simulink model "model_sim_CHB9"  (R2023b)
settings: Solver=FixedStepAuto  StartTime=0.0  StopTime=5  FixedStep=1e-6  RelTol=1e-3
InitFcn:
  | sysinit
values from neighbouring files (symbols this model uses):
  C = 0.0234    [sysinit.m]
  f = 50    [sysinit.m]
  f_switch = 250    [sysinit.m]
  fn = 50    [sysinit.m]
  L = 0.002    [sysinit.m]
  L_ori = 0.02    [sysinit.m]
  L_sec = 0.06    [sysinit.m]
  m = 0.95    [sysinit.m]
  P0 = 8e6    (= 8000000)    [sysinit.m]
  R = 1.5    [sysinit.m]
  Source_Amp = 10000    [sysinit.m]
  st = 1e-6    (= 1e-06)    [sysinit.m]
  Td = 15e-7    (= 1.5e-06)    [sysinit.m]
  Ul_in = 1900    [sysinit.m]
libraries: spsSeriesRLCBranchLib x123, spsDiodeLib x60, spsIGBTLib x48, spsCurrentMeasurementLib x16, spsThreePhaseVIMeasurementLib x13, spsOnDelayLib x12, spsUniversalBridgeLib x12, spsMultiWindingTransformerLib x9, simulink x3, spsVoltageMeasurementLib x3, spsRMSLib x2, spsThreePhaseProgrammableVoltageSourceLib x1
(part 2 of 3)

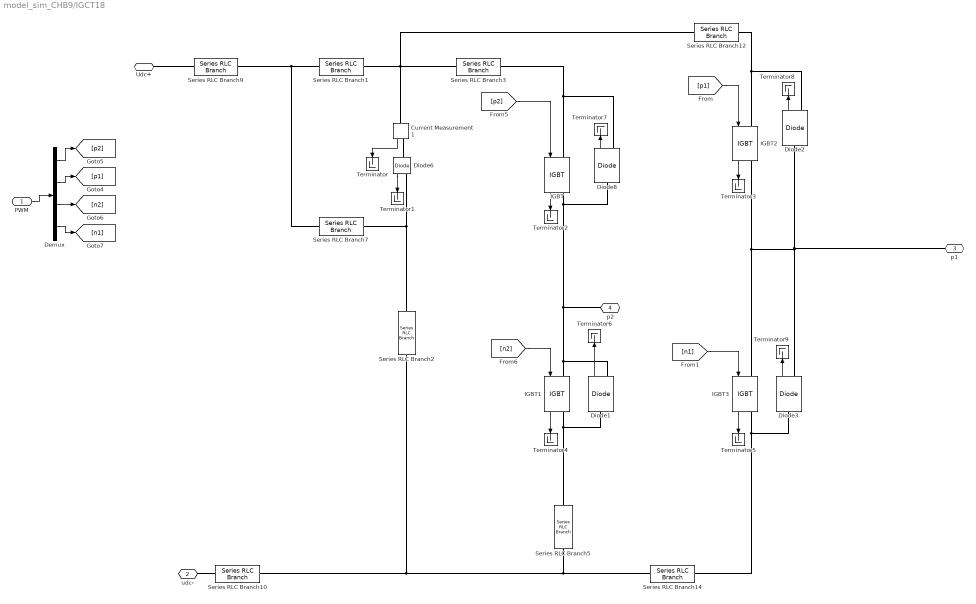
== system model_sim_CHB9/IGCT18 ==
  PWM : Inport
  Current Measurement1 : spsCurrentMeasurementLib/Current Measurement  PhasorSimulation=off  OutputType=Complex  PSBequivalent=0
  Demux : Demux
  Diode{1..3,6,8} (5 alike) : spsDiodeLib/Diode  Ron=rto  Lon=0  Vf=vto  IC=0  UseSnubber=off  Rs=500  Cs=250e-9  Measurements=on
  IGBT{,1..3} (4 alike) : spsIGBTLib/IGBT  Ron=rt  Lon=0  Vf=vt  Tf=1e-6  Tt=2e-6  IC=0  Rs=1e5  Cs=inf  Measurements=on
  Series RLC Branch1 : spsSeriesRLCBranchLib/Series RLC Branch  LConnTagsString=__new0  RConnTagsString=__new0  BranchType=RL  Resistance=1e-5  Inductance=3.0E-6  SetiL0=off  InitialCurrent=0  Capacitance=1e-6  Setx0=off  InitialVoltage=0  Measurements=None
  Series RLC Branch10 : spsSeriesRLCBranchLib/Series RLC Branch  LConnTagsString=__new0  RConnTagsString=__new0  BranchType=L  Resistance=1  Inductance=0.4e-6  SetiL0=off  InitialCurrent=0  Capacitance=1e-6  Setx0=off  InitialVoltage=0  Measurements=None
  Series RLC Branch12 : spsSeriesRLCBranchLib/Series RLC Branch  LConnTagsString=__new0  RConnTagsString=__new0  BranchType=RL  Resistance=1e-5  Inductance=1E-9  SetiL0=off  InitialCurrent=0  Capacitance=1e-6  Setx0=off  InitialVoltage=0  Measurements=None
  Series RLC Branch14 : spsSeriesRLCBranchLib/Series RLC Branch  LConnTagsString=__new0  RConnTagsString=__new0  BranchType=L  Resistance=1  Inductance=1E-7  SetiL0=off  InitialCurrent=0  Capacitance=1e-6  Setx0=off  InitialVoltage=0  Measurements=None
  Series RLC Branch2 : spsSeriesRLCBranchLib/Series RLC Branch  LConnTagsString=__new0  RConnTagsString=__new0  BranchType=RC  Resistance=1e-5  Inductance=20e-6  SetiL0=off  InitialCurrent=0  Capacitance=17e-6  Setx0=off  InitialVoltage=0  Measurements=None
  Series RLC Branch3 : spsSeriesRLCBranchLib/Series RLC Branch  LConnTagsString=__new0  RConnTagsString=__new0  BranchType=RL  Resistance=1e-5  Inductance=1E-9  SetiL0=off  InitialCurrent=0  Capacitance=1e-6  Setx0=off  InitialVoltage=0  Measurements=None
  Series RLC Branch5 : spsSeriesRLCBranchLib/Series RLC Branch  LConnTagsString=__new0  RConnTagsString=__new0  BranchType=L  Resistance=1  Inductance=1E-7  SetiL0=off  InitialCurrent=0  Capacitance=1e-6  Setx0=off  InitialVoltage=0  Measurements=None
  Series RLC Branch7 : spsSeriesRLCBranchLib/Series RLC Branch  LConnTagsString=__new0  RConnTagsString=__new0  BranchType=RL  Resistance=0.6  Inductance=1e-6  SetiL0=off  InitialCurrent=0  Capacitance=1e-6  Setx0=off  InitialVoltage=0  Measurements=None
  Series RLC Branch9 : spsSeriesRLCBranchLib/Series RLC Branch  LConnTagsString=__new0  RConnTagsString=__new0  BranchType=L  Resistance=1  Inductance=0.4e-6  SetiL0=off  InitialCurrent=0  Capacitance=1e-6  Setx0=off  InitialVoltage=0  Measurements=None
  Terminator{,1..9} (10 alike) : Terminator
  Udc+ : PMIOPort  Side=Left
  udc- : PMIOPort  Port=2  Side=Left
  p1 : PMIOPort  Port=3  Side=Right
  p2 : PMIOPort  Port=4  Side=Right
  wires:
  Diode3/1 -> Terminator9/1
  IGBT3/1 -> Terminator5/1
  [n1] -> IGBT3/1
  IGBT1/1 -> Terminator4/1
  IGBT2/1 -> Terminator3/1
  IGBT/1 -> Terminator2/1
  [n2] -> IGBT1/1
  [p1] -> IGBT2/1
  Current Measurement1/1 -> Terminator/1
  Diode2/1 -> Terminator8/1
  [p2] -> IGBT/1
  Diode8/1 -> Terminator7/1
  Diode1/1 -> Terminator6/1
  Diode6/1 -> Terminator1/1
  Demux/3 -> [n2]
  PWM/1 -> Demux/1
  Demux/1 -> [p2]
  Demux/2 -> [p1]
  Demux/4 -> [n1]
  connections:
  Series RLC Branch10/LConn1 -- udc-/RConn1
  Series RLC Branch9/LConn1 -- Udc+/RConn1
  Diode6/RConn1 -- Series RLC Branch7/RConn1 -- Series RLC Branch2/LConn1
  Current Measurement1/LConn1 -- Series RLC Branch1/RConn1 -- Series RLC Branch3/LConn1 -- Series RLC Branch12/LConn1
  Diode3/LConn1 -- IGBT3/RConn1 -- Series RLC Branch14/RConn1
  Series RLC Branch3/RConn1 -- IGBT/LConn1 -- Diode8/RConn1
  Diode1/LConn1 -- Series RLC Branch5/RConn1 -- IGBT1/RConn1
  Current Measurement1/RConn1 -- Diode6/LConn1
  Diode2/RConn1 -- Series RLC Branch12/RConn1 -- IGBT2/LConn1
  p1/RConn1 -- Diode2/LConn1 -- Diode3/RConn1 -- IGBT3/LConn1 -- IGBT2/RConn1
  Series RLC Branch5/LConn1 -- Series RLC Branch14/LConn1 -- Series RLC Branch10/RConn1 -- Series RLC Branch2/RConn1
  Series RLC Branch1/LConn1 -- Series RLC Branch7/LConn1 -- Series RLC Branch9/RConn1
  p2/RConn1 -- IGBT1/LConn1 -- Diode1/RConn1 -- Diode8/LConn1 -- IGBT/RConn1

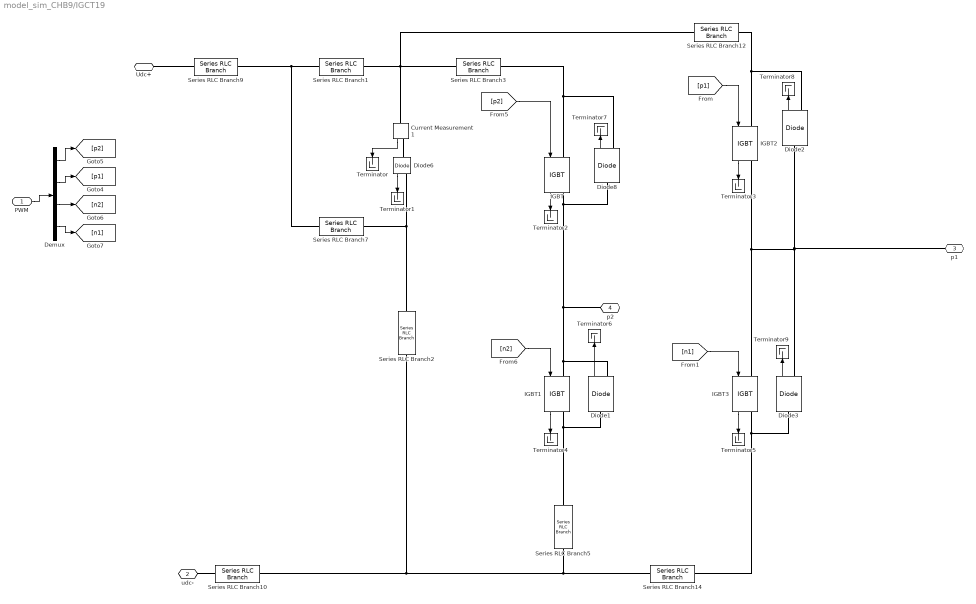
== system model_sim_CHB9/IGCT19 ==
  PWM : Inport
  Current Measurement1 : spsCurrentMeasurementLib/Current Measurement  PhasorSimulation=off  OutputType=Complex  PSBequivalent=0
  Demux : Demux
  Diode{1..3,6,8} (5 alike) : spsDiodeLib/Diode  Ron=rto  Lon=0  Vf=vto  IC=0  UseSnubber=off  Rs=500  Cs=250e-9  Measurements=on
  IGBT{,1..3} (4 alike) : spsIGBTLib/IGBT  Ron=rt  Lon=0  Vf=vt  Tf=1e-6  Tt=2e-6  IC=0  Rs=1e5  Cs=inf  Measurements=on
  Series RLC Branch1 : spsSeriesRLCBranchLib/Series RLC Branch  LConnTagsString=__new0  RConnTagsString=__new0  BranchType=RL  Resistance=1e-5  Inductance=3.0E-6  SetiL0=off  InitialCurrent=0  Capacitance=1e-6  Setx0=off  InitialVoltage=0  Measurements=None
  Series RLC Branch10 : spsSeriesRLCBranchLib/Series RLC Branch  LConnTagsString=__new0  RConnTagsString=__new0  BranchType=L  Resistance=1  Inductance=0.4e-6  SetiL0=off  InitialCurrent=0  Capacitance=1e-6  Setx0=off  InitialVoltage=0  Measurements=None
  Series RLC Branch12 : spsSeriesRLCBranchLib/Series RLC Branch  LConnTagsString=__new0  RConnTagsString=__new0  BranchType=RL  Resistance=1e-5  Inductance=1E-9  SetiL0=off  InitialCurrent=0  Capacitance=1e-6  Setx0=off  InitialVoltage=0  Measurements=None
  Series RLC Branch14 : spsSeriesRLCBranchLib/Series RLC Branch  LConnTagsString=__new0  RConnTagsString=__new0  BranchType=L  Resistance=1  Inductance=1E-7  SetiL0=off  InitialCurrent=0  Capacitance=1e-6  Setx0=off  InitialVoltage=0  Measurements=None
  Series RLC Branch2 : spsSeriesRLCBranchLib/Series RLC Branch  LConnTagsString=__new0  RConnTagsString=__new0  BranchType=RC  Resistance=1e-5  Inductance=20e-6  SetiL0=off  InitialCurrent=0  Capacitance=17e-6  Setx0=off  InitialVoltage=0  Measurements=None
  Series RLC Branch3 : spsSeriesRLCBranchLib/Series RLC Branch  LConnTagsString=__new0  RConnTagsString=__new0  BranchType=RL  Resistance=1e-5  Inductance=1E-9  SetiL0=off  InitialCurrent=0  Capacitance=1e-6  Setx0=off  InitialVoltage=0  Measurements=None
  Series RLC Branch5 : spsSeriesRLCBranchLib/Series RLC Branch  LConnTagsString=__new0  RConnTagsString=__new0  BranchType=L  Resistance=1  Inductance=1E-7  SetiL0=off  InitialCurrent=0  Capacitance=1e-6  Setx0=off  InitialVoltage=0  Measurements=None
  Series RLC Branch7 : spsSeriesRLCBranchLib/Series RLC Branch  LConnTagsString=__new0  RConnTagsString=__new0  BranchType=RL  Resistance=0.6  Inductance=1e-6  SetiL0=off  InitialCurrent=0  Capacitance=1e-6  Setx0=off  InitialVoltage=0  Measurements=None
  Series RLC Branch9 : spsSeriesRLCBranchLib/Series RLC Branch  LConnTagsString=__new0  RConnTagsString=__new0  BranchType=L  Resistance=1  Inductance=0.4e-6  SetiL0=off  InitialCurrent=0  Capacitance=1e-6  Setx0=off  InitialVoltage=0  Measurements=None
  Terminator{,1..9} (10 alike) : Terminator
  Udc+ : PMIOPort  Side=Left
  udc- : PMIOPort  Port=2  Side=Left
  p1 : PMIOPort  Port=3  Side=Right
  p2 : PMIOPort  Port=4  Side=Right
  wires:
  Diode3/1 -> Terminator9/1
  IGBT3/1 -> Terminator5/1
  [n1] -> IGBT3/1
  IGBT1/1 -> Terminator4/1
  IGBT2/1 -> Terminator3/1
  IGBT/1 -> Terminator2/1
  [n2] -> IGBT1/1
  [p1] -> IGBT2/1
  Current Measurement1/1 -> Terminator/1
  Diode2/1 -> Terminator8/1
  [p2] -> IGBT/1
  Diode8/1 -> Terminator7/1
  Diode1/1 -> Terminator6/1
  Diode6/1 -> Terminator1/1
  Demux/3 -> [n2]
  PWM/1 -> Demux/1
  Demux/1 -> [p2]
  Demux/2 -> [p1]
  Demux/4 -> [n1]
  connections:
  Series RLC Branch10/LConn1 -- udc-/RConn1
  Series RLC Branch9/LConn1 -- Udc+/RConn1
  Diode6/RConn1 -- Series RLC Branch7/RConn1 -- Series RLC Branch2/LConn1
  Current Measurement1/LConn1 -- Series RLC Branch1/RConn1 -- Series RLC Branch3/LConn1 -- Series RLC Branch12/LConn1
  Diode3/LConn1 -- IGBT3/RConn1 -- Series RLC Branch14/RConn1
  Series RLC Branch3/RConn1 -- IGBT/LConn1 -- Diode8/RConn1
  Diode1/LConn1 -- Series RLC Branch5/RConn1 -- IGBT1/RConn1
  Current Measurement1/RConn1 -- Diode6/LConn1
  Diode2/RConn1 -- Series RLC Branch12/RConn1 -- IGBT2/LConn1
  p1/RConn1 -- Diode2/LConn1 -- Diode3/RConn1 -- IGBT3/LConn1 -- IGBT2/RConn1
  Series RLC Branch5/LConn1 -- Series RLC Branch14/LConn1 -- Series RLC Branch10/RConn1 -- Series RLC Branch2/RConn1
  Series RLC Branch1/LConn1 -- Series RLC Branch7/LConn1 -- Series RLC Branch9/RConn1
  p2/RConn1 -- IGBT1/LConn1 -- Diode1/RConn1 -- Diode8/LConn1 -- IGBT/RConn1

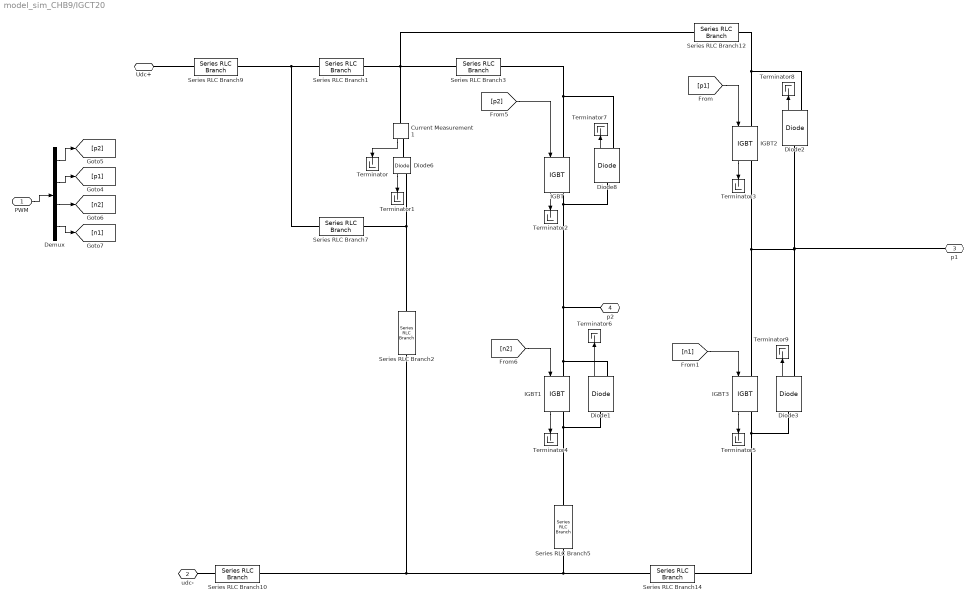
== system model_sim_CHB9/IGCT20 ==
  PWM : Inport
  Current Measurement1 : spsCurrentMeasurementLib/Current Measurement  PhasorSimulation=off  OutputType=Complex  PSBequivalent=0
  Demux : Demux
  Diode{1..3,6,8} (5 alike) : spsDiodeLib/Diode  Ron=rto  Lon=0  Vf=vto  IC=0  UseSnubber=off  Rs=500  Cs=250e-9  Measurements=on
  IGBT{,1..3} (4 alike) : spsIGBTLib/IGBT  Ron=rt  Lon=0  Vf=vt  Tf=1e-6  Tt=2e-6  IC=0  Rs=1e5  Cs=inf  Measurements=on
  Series RLC Branch1 : spsSeriesRLCBranchLib/Series RLC Branch  LConnTagsString=__new0  RConnTagsString=__new0  BranchType=RL  Resistance=1e-5  Inductance=3.0E-6  SetiL0=off  InitialCurrent=0  Capacitance=1e-6  Setx0=off  InitialVoltage=0  Measurements=None
  Series RLC Branch10 : spsSeriesRLCBranchLib/Series RLC Branch  LConnTagsString=__new0  RConnTagsString=__new0  BranchType=L  Resistance=1  Inductance=0.4e-6  SetiL0=off  InitialCurrent=0  Capacitance=1e-6  Setx0=off  InitialVoltage=0  Measurements=None
  Series RLC Branch12 : spsSeriesRLCBranchLib/Series RLC Branch  LConnTagsString=__new0  RConnTagsString=__new0  BranchType=RL  Resistance=1e-5  Inductance=1E-9  SetiL0=off  InitialCurrent=0  Capacitance=1e-6  Setx0=off  InitialVoltage=0  Measurements=None
  Series RLC Branch14 : spsSeriesRLCBranchLib/Series RLC Branch  LConnTagsString=__new0  RConnTagsString=__new0  BranchType=L  Resistance=1  Inductance=1E-7  SetiL0=off  InitialCurrent=0  Capacitance=1e-6  Setx0=off  InitialVoltage=0  Measurements=None
  Series RLC Branch2 : spsSeriesRLCBranchLib/Series RLC Branch  LConnTagsString=__new0  RConnTagsString=__new0  BranchType=RC  Resistance=1e-5  Inductance=20e-6  SetiL0=off  InitialCurrent=0  Capacitance=17e-6  Setx0=off  InitialVoltage=0  Measurements=None
  Series RLC Branch3 : spsSeriesRLCBranchLib/Series RLC Branch  LConnTagsString=__new0  RConnTagsString=__new0  BranchType=RL  Resistance=1e-5  Inductance=1E-9  SetiL0=off  InitialCurrent=0  Capacitance=1e-6  Setx0=off  InitialVoltage=0  Measurements=None
  Series RLC Branch5 : spsSeriesRLCBranchLib/Series RLC Branch  LConnTagsString=__new0  RConnTagsString=__new0  BranchType=L  Resistance=1  Inductance=1E-7  SetiL0=off  InitialCurrent=0  Capacitance=1e-6  Setx0=off  InitialVoltage=0  Measurements=None
  Series RLC Branch7 : spsSeriesRLCBranchLib/Series RLC Branch  LConnTagsString=__new0  RConnTagsString=__new0  BranchType=RL  Resistance=0.6  Inductance=1e-6  SetiL0=off  InitialCurrent=0  Capacitance=1e-6  Setx0=off  InitialVoltage=0  Measurements=None
  Series RLC Branch9 : spsSeriesRLCBranchLib/Series RLC Branch  LConnTagsString=__new0  RConnTagsString=__new0  BranchType=L  Resistance=1  Inductance=0.4e-6  SetiL0=off  InitialCurrent=0  Capacitance=1e-6  Setx0=off  InitialVoltage=0  Measurements=None
  Terminator{,1..9} (10 alike) : Terminator
  Udc+ : PMIOPort  Side=Left
  udc- : PMIOPort  Port=2  Side=Left
  p1 : PMIOPort  Port=3  Side=Right
  p2 : PMIOPort  Port=4  Side=Right
  wires:
  Diode3/1 -> Terminator9/1
  IGBT3/1 -> Terminator5/1
  [n1] -> IGBT3/1
  IGBT1/1 -> Terminator4/1
  IGBT2/1 -> Terminator3/1
  IGBT/1 -> Terminator2/1
  [n2] -> IGBT1/1
  [p1] -> IGBT2/1
  Current Measurement1/1 -> Terminator/1
  Diode2/1 -> Terminator8/1
  [p2] -> IGBT/1
  Diode8/1 -> Terminator7/1
  Diode1/1 -> Terminator6/1
  Diode6/1 -> Terminator1/1
  Demux/3 -> [n2]
  PWM/1 -> Demux/1
  Demux/1 -> [p2]
  Demux/2 -> [p1]
  Demux/4 -> [n1]
  connections:
  Series RLC Branch10/LConn1 -- udc-/RConn1
  Series RLC Branch9/LConn1 -- Udc+/RConn1
  Diode6/RConn1 -- Series RLC Branch7/RConn1 -- Series RLC Branch2/LConn1
  Current Measurement1/LConn1 -- Series RLC Branch1/RConn1 -- Series RLC Branch3/LConn1 -- Series RLC Branch12/LConn1
  Diode3/LConn1 -- IGBT3/RConn1 -- Series RLC Branch14/RConn1
  Series RLC Branch3/RConn1 -- IGBT/LConn1 -- Diode8/RConn1
  Diode1/LConn1 -- Series RLC Branch5/RConn1 -- IGBT1/RConn1
  Current Measurement1/RConn1 -- Diode6/LConn1
  Diode2/RConn1 -- Series RLC Branch12/RConn1 -- IGBT2/LConn1
  p1/RConn1 -- Diode2/LConn1 -- Diode3/RConn1 -- IGBT3/LConn1 -- IGBT2/RConn1
  Series RLC Branch5/LConn1 -- Series RLC Branch14/LConn1 -- Series RLC Branch10/RConn1 -- Series RLC Branch2/RConn1
  Series RLC Branch1/LConn1 -- Series RLC Branch7/LConn1 -- Series RLC Branch9/RConn1
  p2/RConn1 -- IGBT1/LConn1 -- Diode1/RConn1 -- Diode8/LConn1 -- IGBT/RConn1

== system model_sim_CHB9/IGCT21 ==
  PWM : Inport
  Current Measurement1 : spsCurrentMeasurementLib/Current Measurement  PhasorSimulation=off  OutputType=Complex  PSBequivalent=0
  Demux : Demux
  Diode{1..3,6,8} (5 alike) : spsDiodeLib/Diode  Ron=rto  Lon=0  Vf=vto  IC=0  UseSnubber=off  Rs=500  Cs=250e-9  Measurements=on
  IGBT{,1..3} (4 alike) : spsIGBTLib/IGBT  Ron=rt  Lon=0  Vf=vt  Tf=1e-6  Tt=2e-6  IC=0  Rs=1e5  Cs=inf  Measurements=on
  Series RLC Branch1 : spsSeriesRLCBranchLib/Series RLC Branch  LConnTagsString=__new0  RConnTagsString=__new0  BranchType=RL  Resistance=1e-5  Inductance=3.0E-6  SetiL0=off  InitialCurrent=0  Capacitance=1e-6  Setx0=off  InitialVoltage=0  Measurements=None
  Series RLC Branch10 : spsSeriesRLCBranchLib/Series RLC Branch  LConnTagsString=__new0  RConnTagsString=__new0  BranchType=L  Resistance=1  Inductance=0.4e-6  SetiL0=off  InitialCurrent=0  Capacitance=1e-6  Setx0=off  InitialVoltage=0  Measurements=None
  Series RLC Branch12 : spsSeriesRLCBranchLib/Series RLC Branch  LConnTagsString=__new0  RConnTagsString=__new0  BranchType=RL  Resistance=1e-5  Inductance=1E-9  SetiL0=off  InitialCurrent=0  Capacitance=1e-6  Setx0=off  InitialVoltage=0  Measurements=None
  Series RLC Branch14 : spsSeriesRLCBranchLib/Series RLC Branch  LConnTagsString=__new0  RConnTagsString=__new0  BranchType=L  Resistance=1  Inductance=1E-7  SetiL0=off  InitialCurrent=0  Capacitance=1e-6  Setx0=off  InitialVoltage=0  Measurements=None
  Series RLC Branch2 : spsSeriesRLCBranchLib/Series RLC Branch  LConnTagsString=__new0  RConnTagsString=__new0  BranchType=RC  Resistance=1e-5  Inductance=20e-6  SetiL0=off  InitialCurrent=0  Capacitance=17e-6  Setx0=off  InitialVoltage=0  Measurements=None
  Series RLC Branch3 : spsSeriesRLCBranchLib/Series RLC Branch  LConnTagsString=__new0  RConnTagsString=__new0  BranchType=RL  Resistance=1e-5  Inductance=1E-9  SetiL0=off  InitialCurrent=0  Capacitance=1e-6  Setx0=off  InitialVoltage=0  Measurements=None
  Series RLC Branch5 : spsSeriesRLCBranchLib/Series RLC Branch  LConnTagsString=__new0  RConnTagsString=__new0  BranchType=L  Resistance=1  Inductance=1E-7  SetiL0=off  InitialCurrent=0  Capacitance=1e-6  Setx0=off  InitialVoltage=0  Measurements=None
  Series RLC Branch7 : spsSeriesRLCBranchLib/Series RLC Branch  LConnTagsString=__new0  RConnTagsString=__new0  BranchType=RL  Resistance=0.6  Inductance=1e-6  SetiL0=off  InitialCurrent=0  Capacitance=1e-6  Setx0=off  InitialVoltage=0  Measurements=None
  Series RLC Branch9 : spsSeriesRLCBranchLib/Series RLC Branch  LConnTagsString=__new0  RConnTagsString=__new0  BranchType=L  Resistance=1  Inductance=0.4e-6  SetiL0=off  InitialCurrent=0  Capacitance=1e-6  Setx0=off  InitialVoltage=0  Measurements=None
  Terminator{,1..9} (10 alike) : Terminator
  Udc+ : PMIOPort  Side=Left
  udc- : PMIOPort  Port=2  Side=Left
  p1 : PMIOPort  Port=3  Side=Right
  p2 : PMIOPort  Port=4  Side=Right
  wires:
  Diode3/1 -> Terminator9/1
  IGBT3/1 -> Terminator5/1
  [n1] -> IGBT3/1
  IGBT1/1 -> Terminator4/1
  IGBT2/1 -> Terminator3/1
  IGBT/1 -> Terminator2/1
  [n2] -> IGBT1/1
  [p1] -> IGBT2/1
  Current Measurement1/1 -> Terminator/1
  Diode2/1 -> Terminator8/1
  [p2] -> IGBT/1
  Diode8/1 -> Terminator7/1
  Diode1/1 -> Terminator6/1
  Diode6/1 -> Terminator1/1
  Demux/3 -> [n2]
  PWM/1 -> Demux/1
  Demux/1 -> [p2]
  Demux/2 -> [p1]
  Demux/4 -> [n1]
  connections:
  Series RLC Branch10/LConn1 -- udc-/RConn1
  Series RLC Branch9/LConn1 -- Udc+/RConn1
  Diode6/RConn1 -- Series RLC Branch7/RConn1 -- Series RLC Branch2/LConn1
  Current Measurement1/LConn1 -- Series RLC Branch1/RConn1 -- Series RLC Branch3/LConn1 -- Series RLC Branch12/LConn1
  Diode3/LConn1 -- IGBT3/RConn1 -- Series RLC Branch14/RConn1
  Series RLC Branch3/RConn1 -- IGBT/LConn1 -- Diode8/RConn1
  Diode1/LConn1 -- Series RLC Branch5/RConn1 -- IGBT1/RConn1
  Current Measurement1/RConn1 -- Diode6/LConn1
  Diode2/RConn1 -- Series RLC Branch12/RConn1 -- IGBT2/LConn1
  p1/RConn1 -- Diode2/LConn1 -- Diode3/RConn1 -- IGBT3/LConn1 -- IGBT2/RConn1
  Series RLC Branch5/LConn1 -- Series RLC Branch14/LConn1 -- Series RLC Branch10/RConn1 -- Series RLC Branch2/RConn1
  Series RLC Branch1/LConn1 -- Series RLC Branch7/LConn1 -- Series RLC Branch9/RConn1
  p2/RConn1 -- IGBT1/LConn1 -- Diode1/RConn1 -- Diode8/LConn1 -- IGBT/RConn1

== system model_sim_CHB9/IGCT22 ==
  PWM : Inport
  Current Measurement1 : spsCurrentMeasurementLib/Current Measurement  PhasorSimulation=off  OutputType=Complex  PSBequivalent=0
  Demux : Demux
  Diode{1..3,6,8} (5 alike) : spsDiodeLib/Diode  Ron=rto  Lon=0  Vf=vto  IC=0  UseSnubber=off  Rs=500  Cs=250e-9  Measurements=on
  IGBT{,1..3} (4 alike) : spsIGBTLib/IGBT  Ron=rt  Lon=0  Vf=vt  Tf=1e-6  Tt=2e-6  IC=0  Rs=1e5  Cs=inf  Measurements=on
  Series RLC Branch1 : spsSeriesRLCBranchLib/Series RLC Branch  LConnTagsString=__new0  RConnTagsString=__new0  BranchType=RL  Resistance=1e-5  Inductance=3.0E-6  SetiL0=off  InitialCurrent=0  Capacitance=1e-6  Setx0=off  InitialVoltage=0  Measurements=None
  Series RLC Branch10 : spsSeriesRLCBranchLib/Series RLC Branch  LConnTagsString=__new0  RConnTagsString=__new0  BranchType=L  Resistance=1  Inductance=0.4e-6  SetiL0=off  InitialCurrent=0  Capacitance=1e-6  Setx0=off  InitialVoltage=0  Measurements=None
  Series RLC Branch12 : spsSeriesRLCBranchLib/Series RLC Branch  LConnTagsString=__new0  RConnTagsString=__new0  BranchType=RL  Resistance=1e-5  Inductance=1E-9  SetiL0=off  InitialCurrent=0  Capacitance=1e-6  Setx0=off  InitialVoltage=0  Measurements=None
  Series RLC Branch14 : spsSeriesRLCBranchLib/Series RLC Branch  LConnTagsString=__new0  RConnTagsString=__new0  BranchType=L  Resistance=1  Inductance=1E-7  SetiL0=off  InitialCurrent=0  Capacitance=1e-6  Setx0=off  InitialVoltage=0  Measurements=None
  Series RLC Branch2 : spsSeriesRLCBranchLib/Series RLC Branch  LConnTagsString=__new0  RConnTagsString=__new0  BranchType=RC  Resistance=1e-5  Inductance=20e-6  SetiL0=off  InitialCurrent=0  Capacitance=17e-6  Setx0=off  InitialVoltage=0  Measurements=None
  Series RLC Branch3 : spsSeriesRLCBranchLib/Series RLC Branch  LConnTagsString=__new0  RConnTagsString=__new0  BranchType=RL  Resistance=1e-5  Inductance=1E-9  SetiL0=off  InitialCurrent=0  Capacitance=1e-6  Setx0=off  InitialVoltage=0  Measurements=None
  Series RLC Branch5 : spsSeriesRLCBranchLib/Series RLC Branch  LConnTagsString=__new0  RConnTagsString=__new0  BranchType=L  Resistance=1  Inductance=1E-7  SetiL0=off  InitialCurrent=0  Capacitance=1e-6  Setx0=off  InitialVoltage=0  Measurements=None
  Series RLC Branch7 : spsSeriesRLCBranchLib/Series RLC Branch  LConnTagsString=__new0  RConnTagsString=__new0  BranchType=RL  Resistance=0.6  Inductance=1e-6  SetiL0=off  InitialCurrent=0  Capacitance=1e-6  Setx0=off  InitialVoltage=0  Measurements=None
  Series RLC Branch9 : spsSeriesRLCBranchLib/Series RLC Branch  LConnTagsString=__new0  RConnTagsString=__new0  BranchType=L  Resistance=1  Inductance=0.4e-6  SetiL0=off  InitialCurrent=0  Capacitance=1e-6  Setx0=off  InitialVoltage=0  Measurements=None
  Terminator{,1..9} (10 alike) : Terminator
  Udc+ : PMIOPort  Side=Left
  udc- : PMIOPort  Port=2  Side=Left
  p1 : PMIOPort  Port=3  Side=Right
  p2 : PMIOPort  Port=4  Side=Right
  wires:
  Demux/4 -> [n1]
  Demux/2 -> [p1]
  Demux/1 -> [p2]
  PWM/1 -> Demux/1
  Demux/3 -> [n2]
  Diode6/1 -> Terminator1/1
  Diode1/1 -> Terminator6/1
  Diode8/1 -> Terminator7/1
  [p2] -> IGBT/1
  Diode2/1 -> Terminator8/1
  Current Measurement1/1 -> Terminator/1
  [p1] -> IGBT2/1
  [n2] -> IGBT1/1
  IGBT/1 -> Terminator2/1
  IGBT2/1 -> Terminator3/1
  IGBT1/1 -> Terminator4/1
  [n1] -> IGBT3/1
  IGBT3/1 -> Terminator5/1
  Diode3/1 -> Terminator9/1
  connections:
  IGBT/RConn1 -- Diode8/LConn1 -- Diode1/RConn1 -- IGBT1/LConn1 -- p2/RConn1
  Series RLC Branch9/RConn1 -- Series RLC Branch7/LConn1 -- Series RLC Branch1/LConn1
  Series RLC Branch2/RConn1 -- Series RLC Branch10/RConn1 -- Series RLC Branch14/LConn1 -- Series RLC Branch5/LConn1
  IGBT2/RConn1 -- IGBT3/LConn1 -- Diode3/RConn1 -- Diode2/LConn1 -- p1/RConn1
  IGBT2/LConn1 -- Series RLC Branch12/RConn1 -- Diode2/RConn1
  Current Measurement1/RConn1 -- Diode6/LConn1
  IGBT1/RConn1 -- Series RLC Branch5/RConn1 -- Diode1/LConn1
  Diode8/RConn1 -- IGBT/LConn1 -- Series RLC Branch3/RConn1
  Series RLC Branch14/RConn1 -- IGBT3/RConn1 -- Diode3/LConn1
  Series RLC Branch12/LConn1 -- Series RLC Branch3/LConn1 -- Series RLC Branch1/RConn1 -- Current Measurement1/LConn1
  Series RLC Branch2/LConn1 -- Series RLC Branch7/RConn1 -- Diode6/RConn1
  Series RLC Branch9/LConn1 -- Udc+/RConn1
  Series RLC Branch10/LConn1 -- udc-/RConn1

== system model_sim_CHB9/IGCT23 ==
  PWM : Inport
  Current Measurement1 : spsCurrentMeasurementLib/Current Measurement  PhasorSimulation=off  OutputType=Complex  PSBequivalent=0
  Demux : Demux
  Diode{1..3,6,8} (5 alike) : spsDiodeLib/Diode  Ron=rto  Lon=0  Vf=vto  IC=0  UseSnubber=off  Rs=500  Cs=250e-9  Measurements=on
  IGBT{,1..3} (4 alike) : spsIGBTLib/IGBT  Ron=rt  Lon=0  Vf=vt  Tf=1e-6  Tt=2e-6  IC=0  Rs=1e5  Cs=inf  Measurements=on
  Series RLC Branch1 : spsSeriesRLCBranchLib/Series RLC Branch  LConnTagsString=__new0  RConnTagsString=__new0  BranchType=RL  Resistance=1e-5  Inductance=3.0E-6  SetiL0=off  InitialCurrent=0  Capacitance=1e-6  Setx0=off  InitialVoltage=0  Measurements=None
  Series RLC Branch10 : spsSeriesRLCBranchLib/Series RLC Branch  LConnTagsString=__new0  RConnTagsString=__new0  BranchType=L  Resistance=1  Inductance=0.4e-6  SetiL0=off  InitialCurrent=0  Capacitance=1e-6  Setx0=off  InitialVoltage=0  Measurements=None
  Series RLC Branch12 : spsSeriesRLCBranchLib/Series RLC Branch  LConnTagsString=__new0  RConnTagsString=__new0  BranchType=RL  Resistance=1e-5  Inductance=1E-9  SetiL0=off  InitialCurrent=0  Capacitance=1e-6  Setx0=off  InitialVoltage=0  Measurements=None
  Series RLC Branch14 : spsSeriesRLCBranchLib/Series RLC Branch  LConnTagsString=__new0  RConnTagsString=__new0  BranchType=L  Resistance=1  Inductance=1E-7  SetiL0=off  InitialCurrent=0  Capacitance=1e-6  Setx0=off  InitialVoltage=0  Measurements=None
  Series RLC Branch2 : spsSeriesRLCBranchLib/Series RLC Branch  LConnTagsString=__new0  RConnTagsString=__new0  BranchType=RC  Resistance=1e-5  Inductance=20e-6  SetiL0=off  InitialCurrent=0  Capacitance=17e-6  Setx0=off  InitialVoltage=0  Measurements=None
  Series RLC Branch3 : spsSeriesRLCBranchLib/Series RLC Branch  LConnTagsString=__new0  RConnTagsString=__new0  BranchType=RL  Resistance=1e-5  Inductance=1E-9  SetiL0=off  InitialCurrent=0  Capacitance=1e-6  Setx0=off  InitialVoltage=0  Measurements=None
  Series RLC Branch5 : spsSeriesRLCBranchLib/Series RLC Branch  LConnTagsString=__new0  RConnTagsString=__new0  BranchType=L  Resistance=1  Inductance=1E-7  SetiL0=off  InitialCurrent=0  Capacitance=1e-6  Setx0=off  InitialVoltage=0  Measurements=None
  Series RLC Branch7 : spsSeriesRLCBranchLib/Series RLC Branch  LConnTagsString=__new0  RConnTagsString=__new0  BranchType=RL  Resistance=0.6  Inductance=1e-6  SetiL0=off  InitialCurrent=0  Capacitance=1e-6  Setx0=off  InitialVoltage=0  Measurements=None
  Series RLC Branch9 : spsSeriesRLCBranchLib/Series RLC Branch  LConnTagsString=__new0  RConnTagsString=__new0  BranchType=L  Resistance=1  Inductance=0.4e-6  SetiL0=off  InitialCurrent=0  Capacitance=1e-6  Setx0=off  InitialVoltage=0  Measurements=None
  Terminator{,1..9} (10 alike) : Terminator
  Udc+ : PMIOPort  Side=Left
  udc- : PMIOPort  Port=2  Side=Left
  p1 : PMIOPort  Port=3  Side=Right
  p2 : PMIOPort  Port=4  Side=Right
  wires:
  Demux/4 -> [n1]
  Demux/2 -> [p1]
  Demux/1 -> [p2]
  PWM/1 -> Demux/1
  Demux/3 -> [n2]
  Diode6/1 -> Terminator1/1
  Diode1/1 -> Terminator6/1
  Diode8/1 -> Terminator7/1
  [p2] -> IGBT/1
  Diode2/1 -> Terminator8/1
  Current Measurement1/1 -> Terminator/1
  [p1] -> IGBT2/1
  [n2] -> IGBT1/1
  IGBT/1 -> Terminator2/1
  IGBT2/1 -> Terminator3/1
  IGBT1/1 -> Terminator4/1
  [n1] -> IGBT3/1
  IGBT3/1 -> Terminator5/1
  Diode3/1 -> Terminator9/1
  connections:
  IGBT/RConn1 -- Diode8/LConn1 -- Diode1/RConn1 -- IGBT1/LConn1 -- p2/RConn1
  Series RLC Branch9/RConn1 -- Series RLC Branch7/LConn1 -- Series RLC Branch1/LConn1
  Series RLC Branch2/RConn1 -- Series RLC Branch10/RConn1 -- Series RLC Branch14/LConn1 -- Series RLC Branch5/LConn1
  IGBT2/RConn1 -- IGBT3/LConn1 -- Diode3/RConn1 -- Diode2/LConn1 -- p1/RConn1
  IGBT2/LConn1 -- Series RLC Branch12/RConn1 -- Diode2/RConn1
  Current Measurement1/RConn1 -- Diode6/LConn1
  IGBT1/RConn1 -- Series RLC Branch5/RConn1 -- Diode1/LConn1
  Diode8/RConn1 -- IGBT/LConn1 -- Series RLC Branch3/RConn1
  Series RLC Branch14/RConn1 -- IGBT3/RConn1 -- Diode3/LConn1
  Series RLC Branch12/LConn1 -- Series RLC Branch3/LConn1 -- Series RLC Branch1/RConn1 -- Current Measurement1/LConn1
  Series RLC Branch2/LConn1 -- Series RLC Branch7/RConn1 -- Diode6/RConn1
  Series RLC Branch9/LConn1 -- Udc+/RConn1
  Series RLC Branch10/LConn1 -- udc-/RConn1

== system model_sim_CHB9/IGCT24 ==
  PWM : Inport
  Current Measurement1 : spsCurrentMeasurementLib/Current Measurement  PhasorSimulation=off  OutputType=Complex  PSBequivalent=0
  Demux : Demux
  Diode{1..3,6,8} (5 alike) : spsDiodeLib/Diode  Ron=rto  Lon=0  Vf=vto  IC=0  UseSnubber=off  Rs=500  Cs=250e-9  Measurements=on
  IGBT{,1..3} (4 alike) : spsIGBTLib/IGBT  Ron=rt  Lon=0  Vf=vt  Tf=1e-6  Tt=2e-6  IC=0  Rs=1e5  Cs=inf  Measurements=on
  Series RLC Branch1 : spsSeriesRLCBranchLib/Series RLC Branch  LConnTagsString=__new0  RConnTagsString=__new0  BranchType=RL  Resistance=1e-5  Inductance=3.0E-6  SetiL0=off  InitialCurrent=0  Capacitance=1e-6  Setx0=off  InitialVoltage=0  Measurements=None
  Series RLC Branch10 : spsSeriesRLCBranchLib/Series RLC Branch  LConnTagsString=__new0  RConnTagsString=__new0  BranchType=L  Resistance=1  Inductance=0.4e-6  SetiL0=off  InitialCurrent=0  Capacitance=1e-6  Setx0=off  InitialVoltage=0  Measurements=None
  Series RLC Branch12 : spsSeriesRLCBranchLib/Series RLC Branch  LConnTagsString=__new0  RConnTagsString=__new0  BranchType=RL  Resistance=1e-5  Inductance=1E-9  SetiL0=off  InitialCurrent=0  Capacitance=1e-6  Setx0=off  InitialVoltage=0  Measurements=None
  Series RLC Branch14 : spsSeriesRLCBranchLib/Series RLC Branch  LConnTagsString=__new0  RConnTagsString=__new0  BranchType=L  Resistance=1  Inductance=1E-7  SetiL0=off  InitialCurrent=0  Capacitance=1e-6  Setx0=off  InitialVoltage=0  Measurements=None
  Series RLC Branch2 : spsSeriesRLCBranchLib/Series RLC Branch  LConnTagsString=__new0  RConnTagsString=__new0  BranchType=RC  Resistance=1e-5  Inductance=20e-6  SetiL0=off  InitialCurrent=0  Capacitance=17e-6  Setx0=off  InitialVoltage=0  Measurements=None
  Series RLC Branch3 : spsSeriesRLCBranchLib/Series RLC Branch  LConnTagsString=__new0  RConnTagsString=__new0  BranchType=RL  Resistance=1e-5  Inductance=1E-9  SetiL0=off  InitialCurrent=0  Capacitance=1e-6  Setx0=off  InitialVoltage=0  Measurements=None
  Series RLC Branch5 : spsSeriesRLCBranchLib/Series RLC Branch  LConnTagsString=__new0  RConnTagsString=__new0  BranchType=L  Resistance=1  Inductance=1E-7  SetiL0=off  InitialCurrent=0  Capacitance=1e-6  Setx0=off  InitialVoltage=0  Measurements=None
  Series RLC Branch7 : spsSeriesRLCBranchLib/Series RLC Branch  LConnTagsString=__new0  RConnTagsString=__new0  BranchType=RL  Resistance=0.6  Inductance=1e-6  SetiL0=off  InitialCurrent=0  Capacitance=1e-6  Setx0=off  InitialVoltage=0  Measurements=None
  Series RLC Branch9 : spsSeriesRLCBranchLib/Series RLC Branch  LConnTagsString=__new0  RConnTagsString=__new0  BranchType=L  Resistance=1  Inductance=0.4e-6  SetiL0=off  InitialCurrent=0  Capacitance=1e-6  Setx0=off  InitialVoltage=0  Measurements=None
  Terminator{,1..9} (10 alike) : Terminator
  Udc+ : PMIOPort  Side=Left
  udc- : PMIOPort  Port=2  Side=Left
  p1 : PMIOPort  Port=3  Side=Right
  p2 : PMIOPort  Port=4  Side=Right
  wires:
  Demux/4 -> [n1]
  Demux/2 -> [p1]
  Demux/1 -> [p2]
  PWM/1 -> Demux/1
  Demux/3 -> [n2]
  Diode6/1 -> Terminator1/1
  Diode1/1 -> Terminator6/1
  Diode8/1 -> Terminator7/1
  [p2] -> IGBT/1
  Diode2/1 -> Terminator8/1
  Current Measurement1/1 -> Terminator/1
  [p1] -> IGBT2/1
  [n2] -> IGBT1/1
  IGBT/1 -> Terminator2/1
  IGBT2/1 -> Terminator3/1
  IGBT1/1 -> Terminator4/1
  [n1] -> IGBT3/1
  IGBT3/1 -> Terminator5/1
  Diode3/1 -> Terminator9/1
  connections:
  IGBT/RConn1 -- Diode8/LConn1 -- Diode1/RConn1 -- IGBT1/LConn1 -- p2/RConn1
  Series RLC Branch9/RConn1 -- Series RLC Branch7/LConn1 -- Series RLC Branch1/LConn1
  Series RLC Branch2/RConn1 -- Series RLC Branch10/RConn1 -- Series RLC Branch14/LConn1 -- Series RLC Branch5/LConn1
  IGBT2/RConn1 -- IGBT3/LConn1 -- Diode3/RConn1 -- Diode2/LConn1 -- p1/RConn1
  IGBT2/LConn1 -- Series RLC Branch12/RConn1 -- Diode2/RConn1
  Current Measurement1/RConn1 -- Diode6/LConn1
  IGBT1/RConn1 -- Series RLC Branch5/RConn1 -- Diode1/LConn1
  Diode8/RConn1 -- IGBT/LConn1 -- Series RLC Branch3/RConn1
  Series RLC Branch14/RConn1 -- IGBT3/RConn1 -- Diode3/LConn1
  Series RLC Branch12/LConn1 -- Series RLC Branch3/LConn1 -- Series RLC Branch1/RConn1 -- Current Measurement1/LConn1
  Series RLC Branch2/LConn1 -- Series RLC Branch7/RConn1 -- Diode6/RConn1
  Series RLC Branch9/LConn1 -- Udc+/RConn1
  Series RLC Branch10/LConn1 -- udc-/RConn1

== system model_sim_CHB9/LOAD1 ==
  Series RLC Branch1 : spsSeriesRLCBranchLib/Series RLC Branch  LConnTagsString=__new0  RConnTagsString=__new0  BranchType=RL  Resistance=R*2  Inductance=L*2  SetiL0=off  InitialCurrent=0  Capacitance=1e-6  Setx0=off  InitialVoltage=0  Measurements=None
  Series RLC Branch2 : spsSeriesRLCBranchLib/Series RLC Branch  LConnTagsString=__new0  RConnTagsString=__new0  BranchType=RL  Resistance=R*2  Inductance=L*2  SetiL0=off  InitialCurrent=0  Capacitance=1e-6  Setx0=off  InitialVoltage=0  Measurements=None
  Series RLC Branch7 : spsSeriesRLCBranchLib/Series RLC Branch  LConnTagsString=__new0  RConnTagsString=__new0  BranchType=RL  Resistance=R*2  Inductance=L*2  SetiL0=off  InitialCurrent=0  Capacitance=1e-6  Setx0=off  InitialVoltage=0  Measurements=None
  A : PMIOPort  Side=Left
  B : PMIOPort  Port=2  Side=Left
  C : PMIOPort  Port=3  Side=Left
  connections:
  Series RLC Branch7/RConn1 -- Series RLC Branch2/RConn1 -- Series RLC Branch1/RConn1
  Series RLC Branch2/LConn1 -- C/RConn1
  Series RLC Branch7/LConn1 -- A/RConn1
  Series RLC Branch1/LConn1 -- B/RConn1

== system model_sim_CHB9/Subsystem1 ==
  Multi-Winding Transformer10 : spsMultiWindingTransformerLib/Multi-Winding Transformer  LeftWindings=1  RightWindings=6  TappedWindings=no taps  NumberOfTaps=2  SetSaturation=off  Hysteresis=off  DataFile='hysteresis.mat'  Measurements=None  UNITS=pu  NominalPower=[P0 fn]  NominalVoltages="[ Source_Amp  Ul_in 0.366/3.721*Source_Amp*(1-0.366)/0.366 0.366/3.721*Source_Amp Ul_in*sqrt(3) 0.366/3.721*Source_Amp*(1-0.366)/0.366 0.366/3.721*Source_Amp]"  WindingResistances="[ 0.005   0.005 0.005 0.005  0.005  0.005  0.005]"  WindingInductances="[ L_ori*6  L_sec L_sec L_sec L_sec L_sec L_sec]"  Rm=50  Lm=50  Saturation=[ 0,0 ; 0.0024,1.2 ; 1.0,1.52 ]  SpecifyInitialFlux=off  InitialFlux=0  BreakLoop=off  DiscreteSolver=Trapezoidal iterative  DataType=off  TransfoNumber=1
      settings: LibrarySourceBlock=|
      | sps_lib/Power Grid Elements/Multi-Winding
      | Transformer
  Multi-Winding Transformer11 : spsMultiWindingTransformerLib/Multi-Winding Transformer  LeftWindings=1  RightWindings=6  TappedWindings=no taps  NumberOfTaps=2  SetSaturation=off  Hysteresis=off  DataFile='hysteresis.mat'  Measurements=None  UNITS=pu  NominalPower=[P0 fn]  NominalVoltages="[ Source_Amp  Ul_in 0.366/3.721*Source_Amp*(1-0.366)/0.366 0.366/3.721*Source_Amp Ul_in*sqrt(3) 0.366/3.721*Source_Amp*(1-0.366)/0.366 0.366/3.721*Source_Amp]"  WindingResistances="[ 0.005   0.005 0.005 0.005  0.005  0.005  0.005]"  WindingInductances="[ L_ori*6  L_sec L_sec L_sec L_sec L_sec L_sec]"  Rm=50  Lm=50  Saturation=[ 0,0 ; 0.0024,1.2 ; 1.0,1.52 ]  SpecifyInitialFlux=off  InitialFlux=0  BreakLoop=off  DiscreteSolver=Trapezoidal iterative  DataType=off  TransfoNumber=1
      settings: LibrarySourceBlock=|
      | sps_lib/Power Grid Elements/Multi-Winding
      | Transformer
  Multi-Winding Transformer9 : spsMultiWindingTransformerLib/Multi-Winding Transformer  LeftWindings=1  RightWindings=6  TappedWindings=no taps  NumberOfTaps=2  SetSaturation=off  Hysteresis=off  DataFile='hysteresis.mat'  Measurements=None  UNITS=pu  NominalPower=[P0 fn]  NominalVoltages="[ Source_Amp  Ul_in 0.366/3.721*Source_Amp*(1-0.366)/0.366 0.366/3.721*Source_Amp Ul_in*sqrt(3) 0.366/3.721*Source_Amp*(1-0.366)/0.366 0.366/3.721*Source_Amp]"  WindingResistances="[ 0.005   0.005 0.005 0.005  0.005  0.005  0.005]"  WindingInductances=[ L_ori*6 L_sec L_sec L_sec L_sec L_sec L_sec ]/6  Rm=50  Lm=50  Saturation=[ 0,0 ; 0.0024,1.2 ; 1.0,1.52 ]  SpecifyInitialFlux=off  InitialFlux=0  BreakLoop=off  DiscreteSolver=Trapezoidal iterative  DataType=off  TransfoNumber=1
      settings: LibrarySourceBlock=|
      | sps_lib/Power Grid Elements/Multi-Winding
      | Transformer
  1+ : PMIOPort  Side=Left
  1+1 : PMIOPort  Port=2  Side=Left
  1+2 : PMIOPort  Port=3  Side=Left
  p-15a : PMIOPort  Port=4  Side=Right
  p-15b : PMIOPort  Port=5  Side=Right
  p-15c : PMIOPort  Port=6  Side=Right
  p0a : PMIOPort  Port=7  Side=Right
  p0b : PMIOPort  Port=8  Side=Right
  p0c : PMIOPort  Port=9  Side=Right
  p15a : PMIOPort  Port=10  Side=Right
  p15b : PMIOPort  Port=11  Side=Right
  p15c : PMIOPort  Port=12  Side=Right
  p30a : PMIOPort  Port=13  Side=Right
  p30b : PMIOPort  Port=14  Side=Right
  p30c : PMIOPort  Port=15  Side=Right
  connections:
  Multi-Winding Transformer11/LConn1 -- 1+2/RConn1
  p15c/RConn1 -- Multi-Winding Transformer11/RConn11
  p15a/RConn1 -- Multi-Winding Transformer9/RConn11
  p0c/RConn1 -- Multi-Winding Transformer11/RConn1
  Multi-Winding Transformer10/LConn1 -- 1+1/RConn1
  p15b/RConn1 -- Multi-Winding Transformer10/RConn11
  p30b/RConn1 -- Multi-Winding Transformer10/RConn7 -- Multi-Winding Transformer11/RConn8
  p0a/RConn1 -- Multi-Winding Transformer9/RConn1
  Multi-Winding Transformer9/LConn1 -- 1+/RConn1
  Multi-Winding Transformer11/RConn10 -- Multi-Winding Transformer10/RConn12 -- Multi-Winding Transformer10/RConn9
  p30c/RConn1 -- Multi-Winding Transformer11/RConn7 -- Multi-Winding Transformer9/RConn8
  Multi-Winding Transformer9/RConn6 -- Multi-Winding Transformer9/RConn3 -- Multi-Winding Transformer11/RConn4
  p30a/RConn1 -- Multi-Winding Transformer9/RConn7 -- Multi-Winding Transformer10/RConn8
  Multi-Winding Transformer11/RConn6 -- Multi-Winding Transformer10/RConn4 -- Multi-Winding Transformer11/RConn3
  Multi-Winding Transformer10/RConn3 -- Multi-Winding Transformer9/RConn4 -- Multi-Winding Transformer10/RConn6
  Multi-Winding Transformer10/RConn1 -- p0b/RConn1
  Multi-Winding Transformer10/RConn10 -- Multi-Winding Transformer9/RConn9 -- Multi-Winding Transformer9/RConn12
  p-15b/RConn1 -- Multi-Winding Transformer10/RConn5
  p-15c/RConn1 -- Multi-Winding Transformer11/RConn5
  Multi-Winding Transformer9/RConn10 -- Multi-Winding Transformer11/RConn9 -- Multi-Winding Transformer11/RConn12
  p-15a/RConn1 -- Multi-Winding Transformer9/RConn5
  Multi-Winding Transformer9/LConn2 -- Multi-Winding Transformer10/LConn2 -- Multi-Winding Transformer11/LConn2
  Multi-Winding Transformer10/RConn2 -- Multi-Winding Transformer9/RConn2 -- Multi-Winding Transformer11/RConn2

== system model_sim_CHB9/Subsystem2 ==
  Multi-Winding Transformer10 : spsMultiWindingTransformerLib/Multi-Winding Transformer  LeftWindings=1  RightWindings=6  TappedWindings=no taps  NumberOfTaps=2  SetSaturation=off  Hysteresis=off  DataFile='hysteresis.mat'  Measurements=None  UNITS=pu  NominalPower=[P0 fn]  NominalVoltages="[ Source_Amp  Ul_in 0.366/3.721*Source_Amp*(1-0.366)/0.366 0.366/3.721*Source_Amp Ul_in*sqrt(3) 0.366/3.721*Source_Amp*(1-0.366)/0.366 0.366/3.721*Source_Amp]"  WindingResistances="[ 0.005   0.005 0.005 0.005  0.005  0.005  0.005]"  WindingInductances="[ L_ori*6  L_sec L_sec L_sec L_sec L_sec L_sec]"  Rm=50  Lm=50  Saturation=[ 0,0 ; 0.0024,1.2 ; 1.0,1.52 ]  SpecifyInitialFlux=off  InitialFlux=0  BreakLoop=off  DiscreteSolver=Trapezoidal iterative  DataType=off  TransfoNumber=1
      settings: LibrarySourceBlock=|
      | sps_lib/Power Grid Elements/Multi-Winding
      | Transformer
  Multi-Winding Transformer11 : spsMultiWindingTransformerLib/Multi-Winding Transformer  LeftWindings=1  RightWindings=6  TappedWindings=no taps  NumberOfTaps=2  SetSaturation=off  Hysteresis=off  DataFile='hysteresis.mat'  Measurements=None  UNITS=pu  NominalPower=[P0 fn]  NominalVoltages="[ Source_Amp  Ul_in 0.366/3.721*Source_Amp*(1-0.366)/0.366 0.366/3.721*Source_Amp Ul_in*sqrt(3) 0.366/3.721*Source_Amp*(1-0.366)/0.366 0.366/3.721*Source_Amp]"  WindingResistances="[ 0.005   0.005 0.005 0.005  0.005  0.005  0.005]"  WindingInductances="[ L_ori*6  L_sec L_sec L_sec L_sec L_sec L_sec]"  Rm=50  Lm=50  Saturation=[ 0,0 ; 0.0024,1.2 ; 1.0,1.52 ]  SpecifyInitialFlux=off  InitialFlux=0  BreakLoop=off  DiscreteSolver=Trapezoidal iterative  DataType=off  TransfoNumber=1
      settings: LibrarySourceBlock=|
      | sps_lib/Power Grid Elements/Multi-Winding
      | Transformer
  Multi-Winding Transformer9 : spsMultiWindingTransformerLib/Multi-Winding Transformer  LeftWindings=1  RightWindings=6  TappedWindings=no taps  NumberOfTaps=2  SetSaturation=off  Hysteresis=off  DataFile='hysteresis.mat'  Measurements=None  UNITS=pu  NominalPower=[P0 fn]  NominalVoltages="[ Source_Amp  Ul_in 0.366/3.721*Source_Amp*(1-0.366)/0.366 0.366/3.721*Source_Amp Ul_in*sqrt(3) 0.366/3.721*Source_Amp*(1-0.366)/0.366 0.366/3.721*Source_Amp]"  WindingResistances="[ 0.005   0.005 0.005 0.005  0.005  0.005  0.005]"  WindingInductances=[ L_ori*6 L_sec L_sec L_sec L_sec L_sec L_sec ]/6  Rm=50  Lm=50  Saturation=[ 0,0 ; 0.0024,1.2 ; 1.0,1.52 ]  SpecifyInitialFlux=off  InitialFlux=0  BreakLoop=off  DiscreteSolver=Trapezoidal iterative  DataType=off  TransfoNumber=1
      settings: LibrarySourceBlock=|
      | sps_lib/Power Grid Elements/Multi-Winding
      | Transformer
  1+ : PMIOPort  Side=Left
  1+1 : PMIOPort  Port=2  Side=Left
  1+2 : PMIOPort  Port=3  Side=Left
  p-15a : PMIOPort  Port=4  Side=Right
  p-15b : PMIOPort  Port=5  Side=Right
  p-15c : PMIOPort  Port=6  Side=Right
  p0a : PMIOPort  Port=7  Side=Right
  p0b : PMIOPort  Port=8  Side=Right
  p0c : PMIOPort  Port=9  Side=Right
  p15a : PMIOPort  Port=10  Side=Right
  p15b : PMIOPort  Port=11  Side=Right
  p15c : PMIOPort  Port=12  Side=Right
  p30a : PMIOPort  Port=13  Side=Right
  p30b : PMIOPort  Port=14  Side=Right
  p30c : PMIOPort  Port=15  Side=Right
  connections:
  Multi-Winding Transformer11/RConn2 -- Multi-Winding Transformer9/RConn2 -- Multi-Winding Transformer10/RConn2
  Multi-Winding Transformer11/LConn2 -- Multi-Winding Transformer10/LConn2 -- Multi-Winding Transformer9/LConn2
  p-15a/RConn1 -- Multi-Winding Transformer9/RConn5
  Multi-Winding Transformer11/RConn12 -- Multi-Winding Transformer11/RConn9 -- Multi-Winding Transformer9/RConn10
  p-15c/RConn1 -- Multi-Winding Transformer11/RConn5
  p-15b/RConn1 -- Multi-Winding Transformer10/RConn5
  Multi-Winding Transformer9/RConn12 -- Multi-Winding Transformer9/RConn9 -- Multi-Winding Transformer10/RConn10
  Multi-Winding Transformer10/RConn1 -- p0b/RConn1
  Multi-Winding Transformer10/RConn6 -- Multi-Winding Transformer9/RConn4 -- Multi-Winding Transformer10/RConn3
  Multi-Winding Transformer11/RConn3 -- Multi-Winding Transformer10/RConn4 -- Multi-Winding Transformer11/RConn6
  Multi-Winding Transformer10/RConn8 -- Multi-Winding Transformer9/RConn7 -- p30a/RConn1
  Multi-Winding Transformer11/RConn4 -- Multi-Winding Transformer9/RConn3 -- Multi-Winding Transformer9/RConn6
  Multi-Winding Transformer9/RConn8 -- Multi-Winding Transformer11/RConn7 -- p30c/RConn1
  Multi-Winding Transformer10/RConn9 -- Multi-Winding Transformer10/RConn12 -- Multi-Winding Transformer11/RConn10
  Multi-Winding Transformer9/LConn1 -- 1+/RConn1
  p0a/RConn1 -- Multi-Winding Transformer9/RConn1
  Multi-Winding Transformer11/RConn8 -- Multi-Winding Transformer10/RConn7 -- p30b/RConn1
  p15b/RConn1 -- Multi-Winding Transformer10/RConn11
  Multi-Winding Transformer10/LConn1 -- 1+1/RConn1
  p0c/RConn1 -- Multi-Winding Transformer11/RConn1
  p15a/RConn1 -- Multi-Winding Transformer9/RConn11
  p15c/RConn1 -- Multi-Winding Transformer11/RConn11
  Multi-Winding Transformer11/LConn1 -- 1+2/RConn1

== system model_sim_CHB9/Subsystem3 ==
  Multi-Winding Transformer10 : spsMultiWindingTransformerLib/Multi-Winding Transformer  LeftWindings=1  RightWindings=6  TappedWindings=no taps  NumberOfTaps=2  SetSaturation=off  Hysteresis=off  DataFile='hysteresis.mat'  Measurements=None  UNITS=pu  NominalPower=[P0 fn]  NominalVoltages="[ Source_Amp  Ul_in 0.366/3.721*Source_Amp*(1-0.366)/0.366 0.366/3.721*Source_Amp Ul_in*sqrt(3) 0.366/3.721*Source_Amp*(1-0.366)/0.366 0.366/3.721*Source_Amp]"  WindingResistances="[ 0.005   0.005 0.005 0.005  0.005  0.005  0.005]"  WindingInductances="[ L_ori*6  L_sec L_sec L_sec L_sec L_sec L_sec]"  Rm=50  Lm=50  Saturation=[ 0,0 ; 0.0024,1.2 ; 1.0,1.52 ]  SpecifyInitialFlux=off  InitialFlux=0  BreakLoop=off  DiscreteSolver=Trapezoidal iterative  DataType=off  TransfoNumber=1
      settings: LibrarySourceBlock=|
      | sps_lib/Power Grid Elements/Multi-Winding
      | Transformer
  Multi-Winding Transformer11 : spsMultiWindingTransformerLib/Multi-Winding Transformer  LeftWindings=1  RightWindings=6  TappedWindings=no taps  NumberOfTaps=2  SetSaturation=off  Hysteresis=off  DataFile='hysteresis.mat'  Measurements=None  UNITS=pu  NominalPower=[P0 fn]  NominalVoltages="[ Source_Amp  Ul_in 0.366/3.721*Source_Amp*(1-0.366)/0.366 0.366/3.721*Source_Amp Ul_in*sqrt(3) 0.366/3.721*Source_Amp*(1-0.366)/0.366 0.366/3.721*Source_Amp]"  WindingResistances="[ 0.005   0.005 0.005 0.005  0.005  0.005  0.005]"  WindingInductances="[ L_ori*6  L_sec L_sec L_sec L_sec L_sec L_sec]"  Rm=50  Lm=50  Saturation=[ 0,0 ; 0.0024,1.2 ; 1.0,1.52 ]  SpecifyInitialFlux=off  InitialFlux=0  BreakLoop=off  DiscreteSolver=Trapezoidal iterative  DataType=off  TransfoNumber=1
      settings: LibrarySourceBlock=|
      | sps_lib/Power Grid Elements/Multi-Winding
      | Transformer
  Multi-Winding Transformer9 : spsMultiWindingTransformerLib/Multi-Winding Transformer  LeftWindings=1  RightWindings=6  TappedWindings=no taps  NumberOfTaps=2  SetSaturation=off  Hysteresis=off  DataFile='hysteresis.mat'  Measurements=None  UNITS=pu  NominalPower=[P0 fn]  NominalVoltages="[ Source_Amp  Ul_in 0.366/3.721*Source_Amp*(1-0.366)/0.366 0.366/3.721*Source_Amp Ul_in*sqrt(3) 0.366/3.721*Source_Amp*(1-0.366)/0.366 0.366/3.721*Source_Amp]"  WindingResistances="[ 0.005   0.005 0.005 0.005  0.005  0.005  0.005]"  WindingInductances=[ L_ori*6 L_sec L_sec L_sec L_sec L_sec L_sec ]/6  Rm=50  Lm=50  Saturation=[ 0,0 ; 0.0024,1.2 ; 1.0,1.52 ]  SpecifyInitialFlux=off  InitialFlux=0  BreakLoop=off  DiscreteSolver=Trapezoidal iterative  DataType=off  TransfoNumber=1
      settings: LibrarySourceBlock=|
      | sps_lib/Power Grid Elements/Multi-Winding
      | Transformer
  1+ : PMIOPort  Side=Left
  1+1 : PMIOPort  Port=2  Side=Left
  1+2 : PMIOPort  Port=3  Side=Left
  p-15a : PMIOPort  Port=4  Side=Right
  p-15b : PMIOPort  Port=5  Side=Right
  p-15c : PMIOPort  Port=6  Side=Right
  p0a : PMIOPort  Port=7  Side=Right
  p0b : PMIOPort  Port=8  Side=Right
  p0c : PMIOPort  Port=9  Side=Right
  p15a : PMIOPort  Port=10  Side=Right
  p15b : PMIOPort  Port=11  Side=Right
  p15c : PMIOPort  Port=12  Side=Right
  p30a : PMIOPort  Port=13  Side=Right
  p30b : PMIOPort  Port=14  Side=Right
  p30c : PMIOPort  Port=15  Side=Right
  connections:
  Multi-Winding Transformer11/LConn1 -- 1+2/RConn1
  p15c/RConn1 -- Multi-Winding Transformer11/RConn11
  p15a/RConn1 -- Multi-Winding Transformer9/RConn11
  p0c/RConn1 -- Multi-Winding Transformer11/RConn1
  Multi-Winding Transformer10/LConn1 -- 1+1/RConn1
  p15b/RConn1 -- Multi-Winding Transformer10/RConn11
  p30b/RConn1 -- Multi-Winding Transformer10/RConn7 -- Multi-Winding Transformer11/RConn8
  p0a/RConn1 -- Multi-Winding Transformer9/RConn1
  Multi-Winding Transformer9/LConn1 -- 1+/RConn1
  Multi-Winding Transformer11/RConn10 -- Multi-Winding Transformer10/RConn12 -- Multi-Winding Transformer10/RConn9
  p30c/RConn1 -- Multi-Winding Transformer11/RConn7 -- Multi-Winding Transformer9/RConn8
  Multi-Winding Transformer9/RConn6 -- Multi-Winding Transformer9/RConn3 -- Multi-Winding Transformer11/RConn4
  p30a/RConn1 -- Multi-Winding Transformer9/RConn7 -- Multi-Winding Transformer10/RConn8
  Multi-Winding Transformer11/RConn6 -- Multi-Winding Transformer10/RConn4 -- Multi-Winding Transformer11/RConn3
  Multi-Winding Transformer10/RConn3 -- Multi-Winding Transformer9/RConn4 -- Multi-Winding Transformer10/RConn6
  Multi-Winding Transformer10/RConn1 -- p0b/RConn1
  Multi-Winding Transformer10/RConn10 -- Multi-Winding Transformer9/RConn9 -- Multi-Winding Transformer9/RConn12
  p-15b/RConn1 -- Multi-Winding Transformer10/RConn5
  p-15c/RConn1 -- Multi-Winding Transformer11/RConn5
  Multi-Winding Transformer9/RConn10 -- Multi-Winding Transformer11/RConn9 -- Multi-Winding Transformer11/RConn12
  p-15a/RConn1 -- Multi-Winding Transformer9/RConn5
  Multi-Winding Transformer9/LConn2 -- Multi-Winding Transformer10/LConn2 -- Multi-Winding Transformer11/LConn2
  Multi-Winding Transformer10/RConn2 -- Multi-Winding Transformer9/RConn2 -- Multi-Winding Transformer11/RConn2

== system model_sim_CHB9/Subsystem4 ==
  Current Measurement : spsCurrentMeasurementLib/Current Measurement  PhasorSimulation=off  OutputType=Complex  PSBequivalent=0
  Voltage Measurement : spsVoltageMeasurementLib/Voltage Measurement  PhasorSimulation=off  OutputType=Complex  PSBequivalent=0
  + : PMIOPort  Side=Left
  - : PMIOPort  Port=2  Side=Left
  +OUT : PMIOPort  Port=3  Side=Right
  -OUT : PMIOPort  Port=4  Side=Right
  tag scope: Idc=global, Udc=global
  wires:
  Current Measurement/1 -> [Idc]
  Voltage Measurement/1 -> [Udc]
  connections:
  Current Measurement/RConn1 -- +OUT/RConn1
  -/RConn1 -- -OUT/RConn1 -- Voltage Measurement/LConn2
  +/RConn1 -- Current Measurement/LConn1 -- Voltage Measurement/LConn1
